simulink model "SpeedControl_PWM"  (Simulink 7.4)
settings: Solver=ode1  SolverMode=SingleTasking  StartTime=0.0  StopTime=inf  FixedStep=0.01  MaxStep=0.02  RelTol=1e-3  AbsTol=1e-6
undefined symbols (not defined in the file or in its folder): bit
libraries: simulink_extras x1, mc9s12tool x1
CloseFcn:
  | rtwprivate ssgencode ModelCloseRequest MC_AD
settings Model: Creator=fwornle  LastModifiedBy=fw  SimulationMode=external  ExtModeTrigDuration=800
settings ConfigSet: Description=rtmc9s12target_R2009b
settings DataIOCC: LimitDataPoints=off  SaveOutput=off  SaveTime=off  SignalLoggingName=sigsOut
settings OptimizationCC: BlockReduction=off  BooleanDataType=off  InitFltsAndDblsToZero=on  OptimizeModelRefInitCode=on  LifeSpan=1
settings DebuggingCC: SaveWithParameterizedLinksMsg=none  SignalResolutionControl=TryResolveAllWithWarning  SolverPrmCheckMsg=none  MultiTaskDSMMsg=warning  MultiTaskCondExecSysMsg=none  StrictBusMsg=None
settings HardwareCC: ProdBitPerInt=16  ProdEndianess=BigEndian  ProdWordSize=16  ProdHWDeviceType=Motorola HC12
settings RTWCC: SystemTargetFile=mc9s12.tlc  GenerateMakefile=off  TemplateMakefile=mc9s12.tmf  ProcessScript=mc9s12_make_rtw_hook  IncludeERTFirstTime=on
settings CodeAppCC: IgnoreCustomStorageClasses=off
settings STFCustomTargetCC: TargetFcnLib=ansi_tfl_tmw.mat  ModelReferenceCompliant=off  IncludeMdlTerminateFcn=off  ERTCustomFileBanners=on  SupportNonInlinedSFcns=off  CPPClassGenCompliant=on  SystemTargetFile=mc9s12.tlc
settings ERTTargetCC: TargetFcnLib=ansi_tfl_tmw.mat  MultiwordLength=2048  ModelReferenceCompliant=off  ParMdlRefBuildCompliant=off  CompOptLevelCompliant=off  IncludeMdlTerminateFcn=off  CombineOutputUpdateFcns=off  ERTFirstTimeCompliant=off  SupportContinuousTime=on  ModelStepFunctionPrototypeControlCompliant=off  ExtMode=on  ExtModeMexFile=ext_serial_mc9s12_comm  ExtModeMexArgs=1,2,115200  InlinedParameterPlacement=NonHierarchical  ERTCustomFileTemplate=mc9s12_file_process.tlc  GRTInterface=on  ConvertIfToSwitch=off
settings CustomProperty: DataType=RTWOptions_EnumType_C__Users_fw__SVN_rtmc9s12-target_trunk_rtmc9s12_CW_R2009b_bin_mc9s12_1mc9s12_TargetBoard  Value=Dragon12Plus
settings EnumStrPairs: String=Dragon12

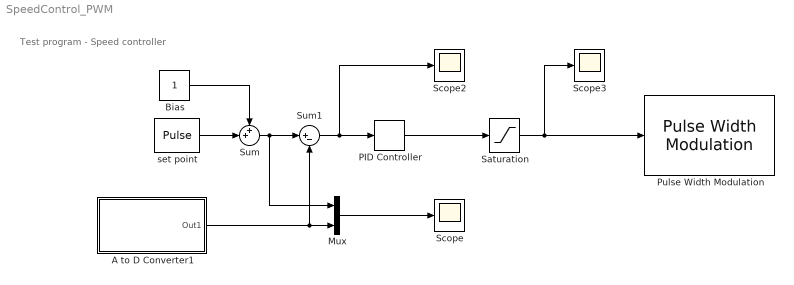
== system SpeedControl_PWM ==
  note: Test program - Speed controller
  A to D Converter1 : Subsystem  Tag=mcTarget_adc  mask{bank=0, channels=3, use10bits=10 bits, normalize=max. output:  5, sampletime=0.01}
      mask prompts: bank "ADC bank"; channels "Channels ( 0 - 7 )"; use10bits "ADC resolution"; normalize "Normalization"; sampletime "Sample time"
      mask init:
      | [channelsStr, firstChannel, numChannels] = mbc_adcinput(channels);
      mask Help: web('adc_sfcn_9S12.html');
      mask StyleString: popup(0|1),edit,popup(10 bits|8 bits),popup(raw values|max. output:  1|max. output:  5),edit
      mask Display: disp(['A to D Converter\n' channelsStr])
  Bias : Constant  OutDataType=sfix(16)  OutScaling=2^0
  Mux : Mux  Inputs=2
  PID Controller : simulink_extras/Additional Linear/PID Controller  SystemSampleTime=-1  P=1.0  I=.2  D=0.00
  Pulse Width Modulation : mc9s12tool/Pulse Width Modulation  Tag=mcTarget_pwm  SystemSampleTime=-1  sampletime=0.01  resolution=16 bit  PWMperiod=0.01  pulse_pin="1  (8-bit / 16-bit)"  sign_port=PTH  sign_pin=1  Vmax=5  sig_mon=off
  Saturation : Saturate  UpperLimit=5  LowerLimit=0
  Scope : Scope
      settings: TimeRange=8  YMin=-0.5  YMax=5.5
  Scope2 : Scope
      settings: TimeRange=8  YMin=-5.5  YMax=5.5  SaveName=ScopeData2
  Scope3 : Scope
      settings: TimeRange=8  YMin=-0.5  YMax=5.5  SaveName=ScopeData3
  Sum : Sum  Inputs=++|  OutDataType=sfix(16)  OutScaling=2^0  SaturateOnIntegerOverflow=on
  Sum1 : Sum  Inputs=|+-  OutDataType=sfix(16)  OutScaling=2^0  SaturateOnIntegerOverflow=on
  set point : DiscretePulseGenerator  PulseType=Time based  Amplitude=4  Period=4  PulseWidth=50  PhaseDelay=0  SampleTime=1
  wires:
  Saturation/1 -> Scope3/1, Pulse Width Modulation/1
  A to D Converter1/1(Out1) -> Mux/2, Sum1/2
  PID Controller/1 -> Saturation/1
  Mux/1 -> Scope/1
  Bias/1 -> Sum/1
  set point/1 -> Sum/2
  Sum/1 -> Sum1/1, Mux/1
  Sum1/1 -> PID Controller/1, Scope2/1

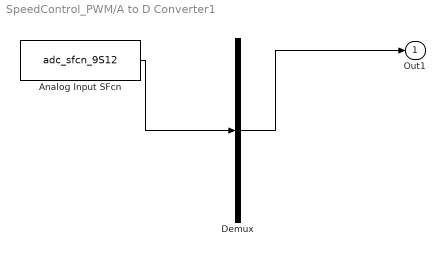
== system SpeedControl_PWM/A to D Converter1 ==
  Analog Input SFcn : S-Function  Tag=mcTarget_adc  FunctionName=adc_sfcn_9S12  Parameters=bank-1, firstChannel, numChannels, use10bits-1, normalize, sampletime  EnableBusSupport=off
  Demux : Demux  Outputs=1
  Out1 : Outport  OutDataType=sfix(16)  OutScaling=2^0
  wires:
  Analog Input SFcn/1 -> Demux/1
  Demux/1 -> Out1/1
